simulink model "ReferencedFlightControlArchitecture"  (R2023b)
settings: Solver=FixedStepDiscrete  StartTime=0.0  StopTime=4  FixedStep=Sample_time  RelTol=1e-3
undefined symbols (not defined in the file): normal_mode_code, Sample_time
libraries: simulink x1
Description:
  | Referenced-model flight-control architecture training example with a typed FlightControlBus and explicit interface routing.
settings Model: DataDictionary=FCS_Data.sldd  Creator=Tyler  LastModifiedBy=Tyler
settings CodeAppCC: MaxIdLength=63

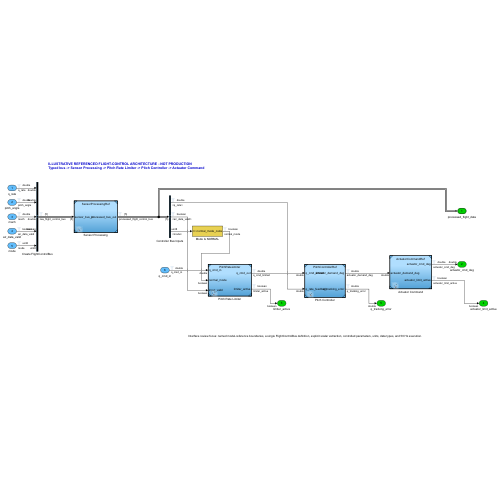
[thumbnail: Simulink's stored preview of the top-level diagram]
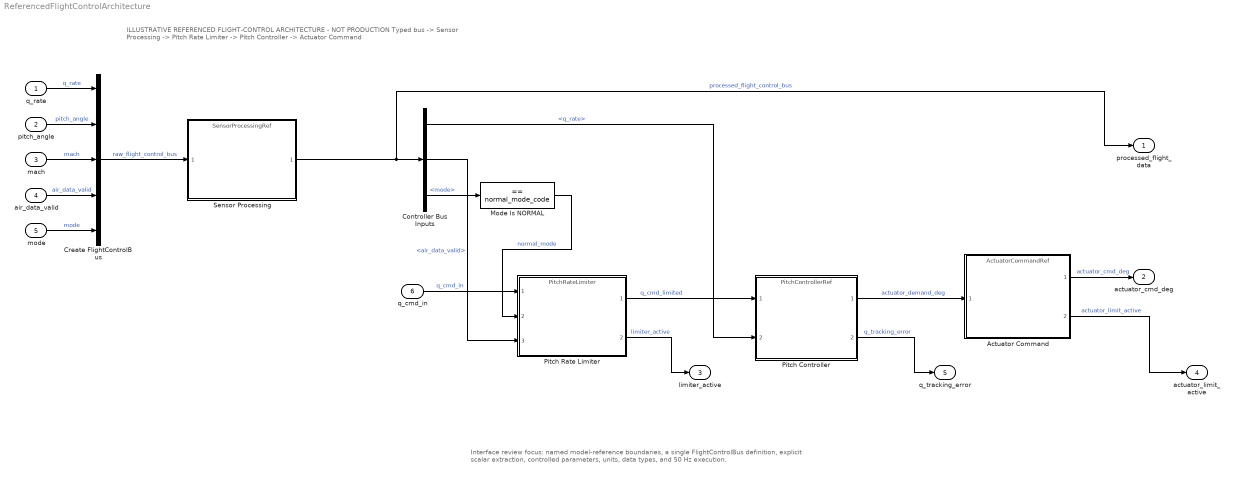
== system ReferencedFlightControlArchitecture ==
  note: ILLUSTRATIVE REFERENCED FLIGHT-CONTROL ARCHITECTURE - NOT PRODUCTION
      | Typed bus -> Sensor Processing -> Pitch Rate Limiter -> Pitch Controller -> Actuator Command
  note: Interface review focus: named model-reference boundaries, a single FlightControlBus definition, explicit scalar extraction, controlled parameters, units, data types, and 50 Hz execution.
  q_rate : Inport  OutDataTypeStr=double  Unit=deg/s  SampleTime=Sample_time
  pitch_angle : Inport  Port=2  OutDataTypeStr=double  Unit=deg  SampleTime=Sample_time
  mach : Inport  Port=3  OutDataTypeStr=double  Unit=1  SampleTime=Sample_time
  air_data_valid : Inport  Port=4  OutDataTypeStr=boolean  Unit=1  SampleTime=Sample_time
  mode : Inport  Port=5  OutDataTypeStr=uint8  Unit=1  SampleTime=Sample_time
  q_cmd_in : Inport  Port=6  OutDataTypeStr=double  Unit=deg/s  SampleTime=Sample_time
  Actuator Command : ModelReference  Description=Model reference to ActuatorCommandRef.slx (illustrative training component).  ModelNameDialog=ActuatorCommandRef  SimulationMode=Accelerator  ModelReferenceVersion=1.2
  Controller Bus Inputs : BusSelector  OutputSignals=q_rate,air_data_valid,mode
  Create FlightControlBus : BusCreator  Inputs=5  OutDataTypeStr=Bus: FlightControlBus
  Mode Is NORMAL : simulink/Logic and Bit Operations/Compare To Constant  relop===  const=normal_mode_code  OutDataTypeStr=boolean
  Pitch Controller : ModelReference  Description=Model reference to PitchControllerRef.slx (illustrative training component).  ModelNameDialog=PitchControllerRef  SimulationMode=Accelerator  ModelReferenceVersion=1.3
  Pitch Rate Limiter : ModelReference  Description=Model reference to PitchRateLimiter.slx (illustrative training component).  ModelNameDialog=PitchRateLimiter  SimulationMode=Accelerator  ModelReferenceVersion=1.2
  Sensor Processing : ModelReference  Description=Model reference to SensorProcessingRef.slx (illustrative training component).  ModelNameDialog=SensorProcessingRef  SimulationMode=Accelerator  ModelReferenceVersion=1.1
  processed_flight_data : Outport  OutDataTypeStr=Bus: FlightControlBus
  actuator_cmd_deg : Outport  Port=2  OutDataTypeStr=double  Unit=deg
  limiter_active : Outport  Port=3  OutDataTypeStr=boolean  Unit=1
  actuator_limit_active : Outport  Port=4  OutDataTypeStr=boolean  Unit=1
  q_tracking_error : Outport  Port=5  OutDataTypeStr=double  Unit=deg/s
  wires:
  q_rate/1 -> Create FlightControlBus/1  "q_rate"
  pitch_angle/1 -> Create FlightControlBus/2  "pitch_angle"
  mach/1 -> Create FlightControlBus/3  "mach"
  air_data_valid/1 -> Create FlightControlBus/4  "air_data_valid"
  mode/1 -> Create FlightControlBus/5  "mode"
  Create FlightControlBus/1 -> Sensor Processing/1  "raw_flight_control_bus"
  Sensor Processing/1 -> Controller Bus Inputs/1, processed_flight_data/1  "processed_flight_control_bus"
  Controller Bus Inputs/3 -> Mode Is NORMAL/1  "<mode>"
  q_cmd_in/1 -> Pitch Rate Limiter/1  "q_cmd_in"
  Mode Is NORMAL/1 -> Pitch Rate Limiter/2  "normal_mode"
  Controller Bus Inputs/2 -> Pitch Rate Limiter/3  "<air_data_valid>"
  Pitch Rate Limiter/1 -> Pitch Controller/1  "q_cmd_limited"
  Controller Bus Inputs/1 -> Pitch Controller/2  "<q_rate>"
  Pitch Controller/1 -> Actuator Command/1  "actuator_demand_deg"
  Actuator Command/1 -> actuator_cmd_deg/1  "actuator_cmd_deg"
  Pitch Rate Limiter/2 -> limiter_active/1  "limiter_active"
  Actuator Command/2 -> actuator_limit_active/1  "actuator_limit_active"
  Pitch Controller/2 -> q_tracking_error/1  "q_tracking_error"
